simulink model "tvc_linear"  (R2018b)
settings: Solver=FixedStepAuto  StartTime=0.0  StopTime=5  FixedStep=0.001  RelTol=1e-3
values from neighbouring files (symbols this model uses):
  Ft = 300    [dynamics_gui.m]    (also in tvc.m)
  I = 3.5    [dynamics_gui.m]    (also in tvc.m)
  Kd = 60    [dynamics_gui.m]    (also in tvc.m = 5)
  Ki = 0    [dynamics_gui.m]    (also in tvc.m)
  Kp = 20    [dynamics_gui.m]    (also in tvc.m = 40)
  theta_d = 0    [tvc.m]
  theta_des = 0    [tvc.m]
  theta_max = 30    [tvc.m]
  x_cm = 1.2    [dynamics_gui.m]    (also in tvc.m)
settings Model: Creator=seant  LastModifiedBy=seant
settings DebuggingCC: LibraryContextMissingDiagnostic=none
settings SFSimCC: SimUseLocalCustomCode=off
settings RTWCC: RTWUseLocalCustomCode=off

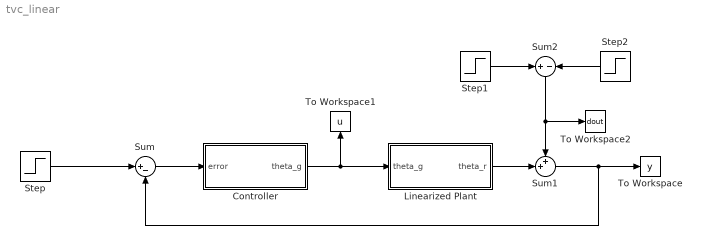
== system tvc_linear ==
  "Controller " : Subsystem
  "Linearized Plant " : Subsystem
  Step : Step  Time=0  After=deg2rad(theta_des)  SampleTime=0
  Step1 : Step  After=deg2rad(theta_d)  SampleTime=0
  Step2 : Step  Time=1.01  After=deg2rad(theta_d)  SampleTime=0
  Sum : Sum  Inputs=|+-
  Sum1 : Sum  Inputs=++|
  Sum2 : Sum  Inputs=+|-
  To Workspace : ToWorkspace  VariableName=y  SaveFormat=Timeseries  SampleTime=-1
  To Workspace1 : ToWorkspace  VariableName=u  SaveFormat=Timeseries  SampleTime=-1
  To Workspace2 : ToWorkspace  VariableName=dout  SaveFormat=Timeseries  SampleTime=-1
  wires:
  Step/1 -> Sum/1
  "Controller "/1(theta_g) -> "Linearized Plant "/1("theta_g "), To Workspace1/1
  Sum/1 -> "Controller "/1(error)
  "Linearized Plant "/1(theta_r) -> Sum1/2
  Sum1/1 -> To Workspace/1, Sum/2
  Step2/1 -> Sum2/2
  Step1/1 -> Sum2/1
  Sum2/1 -> To Workspace2/1, Sum1/1

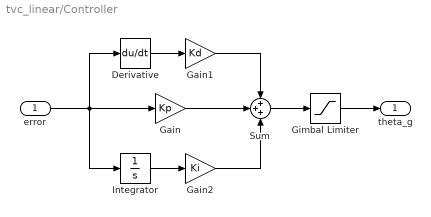
== system tvc_linear/Controller  ==
  error : Inport
  Derivative : Derivative
  Gain : Gain  Gain=Kp
  Gain1 : Gain  Gain=Kd
  Gain2 : Gain  Gain=Ki
  Gimbal Limiter : Saturate  UpperLimit=deg2rad(theta_max)  LowerLimit=-deg2rad(theta_max)
  Integrator : Integrator
  Sum : Sum  Inputs=+++
  theta_g : Outport
  wires:
  error/1 -> Integrator/1, Derivative/1, Gain/1
  Integrator/1 -> Gain2/1
  Derivative/1 -> Gain1/1
  Gain/1 -> Sum/2
  Gain1/1 -> Sum/1
  Gain2/1 -> Sum/3
  Sum/1 -> Gimbal Limiter/1
  Gimbal Limiter/1 -> theta_g/1

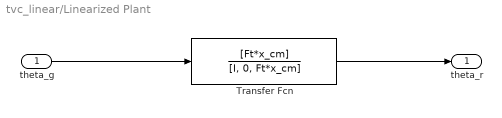
== system tvc_linear/Linearized Plant  ==
  "theta_g " : Inport
  Transfer Fcn : TransferFcn  Numerator=[Ft*x_cm]  Denominator=[I, 0, Ft*x_cm]
  theta_r : Outport
  wires:
  "theta_g "/1 -> Transfer Fcn/1
  Transfer Fcn/1 -> theta_r/1
